simulink model "Teste"  (R2017a)
settings: Solver=FixedStepAuto  StartTime=0.0  StopTime=50  FixedStep=0.1  RelTol=1e-3
values from neighbouring files (symbols this model uses):
  A = [-0.291586,0.,-272.,9.7784;-0.0708916,-2.68243,2.50156,0;0.0200573, -0.0380033,-1.0414,0;0,1,0,0]    [Controlabilidade.m]    (also in Teste_place.m = [-0.291586,0.,-272.,9.7784;-0.0708916,-2.68243,2.50156,0;0.0)
  B1 = [0.291586; 0.0708916; -0.0200573; 0]    [Controlabilidade.m]    (also in Teste_place.m)
  B2 = [0, 10.4276 ;0.932639, 0.745253; -0.0242993, -3.1475; 0, 0]    [Controlabilidade.m]    (also in Teste_place.m)
undefined symbols (not defined in the file or in its folder): B3, p0, phi0, q0, v0
settings Model: Creator=Gabriel  LastModifiedBy=Gabriel

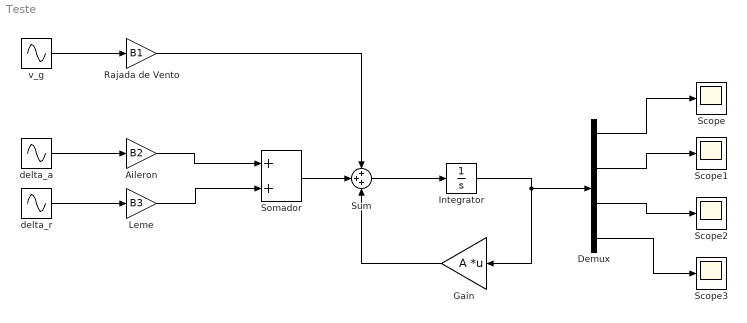
== system Teste ==
  Aileron : Gain  Gain=B2
  Demux : Demux
  Gain : Gain  Gain=A  Multiplication=Matrix(K*u) (u vector)
  Integrator : Integrator  InitialCondition=[v0;p0;q0;phi0]  ZeroCross=off
  Leme : Gain  Gain=B3
  "Rajada de Vento " : Gain  Gain=B1
  Scope{,1..3} (4 alike) : Scope
  "Somador " : Sum  Inputs=2
  Sum : Sum  Inputs=3
  delta_a : Sin  Amplitude=1*pi/180  SampleTime=0
  delta_r : Sin  Amplitude=1*pi/180  SampleTime=0
  v_g : Sin  Amplitude=10  SampleTime=0
  wires:
  Aileron/1 -> "Somador "/1
  Leme/1 -> "Somador "/2
  v_g/1 -> "Rajada de Vento "/1
  delta_r/1 -> Leme/1
  delta_a/1 -> Aileron/1
  Integrator/1 -> Demux/1, Gain/1
  Sum/1 -> Integrator/1
  Gain/1 -> Sum/3
  "Somador "/1 -> Sum/2
  "Rajada de Vento "/1 -> Sum/1
  Demux/1 -> Scope/1
  Demux/2 -> Scope1/1
  Demux/3 -> Scope2/1
  Demux/4 -> Scope3/1
